simulink model "Collision_Test_Block_2020a"  (R2020a)
settings: Solver=ode4  StartTime=0.0  StopTime=15  FixedStep=0.001  RelTol=1e-6
values from neighbouring files (symbols this model uses):
  b = 200000    [Mini_Project.m]
  m = 80000    [Mini_Project.m]
  normal = 9.81*m    (= 784800)    [Mini_Project.m]
  u_kin = 0.05    [Mini_Project.m]
  u_st = 0.15    [Mini_Project.m]
libraries: simulink x3
settings Model: Creator=seano  LastModifiedBy=jackg
settings SolverCC: ZeroCrossAlgorithm=Adaptive
settings DebuggingCC: IgnoredZcDiagnostic=none  SFMachineParentedDataDiag=error

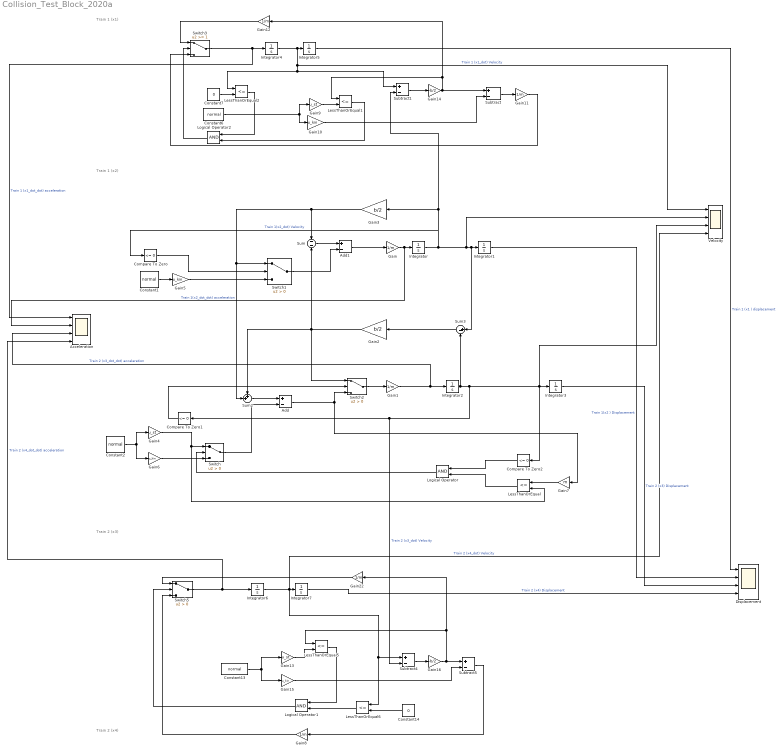
== system Collision_Test_Block_2020a ==
  note: Train 1 (x2)
  note: Train 1 (x1)
  note: Train 2 (x3)
  note: Train 2 (x4)
  Acceleration : Scope  NumInputPorts=4
  Add : Sum  Inputs=+-
  Add1 : Sum  Inputs=+-
  Compare To Zero : simulink/Logic and Bit Operations/Compare To Zero  relop=<=  OutDataTypeStr=boolean
  Compare To Zero1 : simulink/Logic and Bit Operations/Compare To Zero  relop=<=  OutDataTypeStr=boolean
  Compare To Zero2 : simulink/Logic and Bit Operations/Compare To Zero  relop=<=  OutDataTypeStr=boolean
  Constant{1..2,6,13} (4 alike) : Constant  Value=normal
  Constant14 : Constant  Value=0
  Constant7 : Constant  Value=0
  Displacement : Scope  NumInputPorts=4
  Gain{,1,8,11..12,22} (6 alike) : Gain  Gain=1/m
  Gain{5..6,10,15} (4 alike) : Gain  Gain=u_kin
  Gain13 : Gain  Gain=u_st
  Gain14 : Gain  Gain=-b/2
  Gain16 : Gain  Gain=-b/2
  Gain2 : Gain  Gain=b/2
  Gain3 : Gain  Gain=b/2
  Gain4 : Gain  Gain=u_st
  Gain7 : Gain  Gain=m
  Gain9 : Gain  Gain=u_st
  Integrator : Integrator  InitialCondition=13.9
  Integrator{1,3,5,7} (4 alike) : Integrator  InitialCondition=50
  Integrator2 : Integrator
  Integrator4 : Integrator  InitialCondition=13.9
  Integrator6 : Integrator
  LessThanOrEqual{,1..2,5..6} (5 alike) : RelationalOperator  Operator=<=  OutDataTypeStr=boolean  RndMeth=Simplest
  Logical Operator : Logic  AllPortsSameDT=off  OutDataTypeStr=boolean
  Logical Operator1 : Logic  AllPortsSameDT=off  OutDataTypeStr=boolean
  Logical Operator2 : Logic  AllPortsSameDT=off  OutDataTypeStr=boolean
  Subtract{,1,4..5} (4 alike) : Sum  Inputs=+-
  Sum : Sum  Inputs=--
  Sum2 : Sum  Inputs=++|
  Sum3 : Sum  Inputs=|+-
  Switch{,1..2,5} (4 alike) : Switch  Criteria=u2 > Threshold
  Switch3 : Switch  Threshold=1
  Velocity : Scope  NumInputPorts=4
  wires:
  Integrator/1 -> Subtract1/2, Gain3/1, Compare To Zero/1, Sum3/1, Integrator1/1, Velocity/2  "Train 1(x2_dot) Velocity"
  Integrator1/1 -> Displacement/2  "Train 1(x2 ) Displacement"
  Integrator3/1 -> Displacement/3  "Train 2 (x3) Displacement"
  Sum3/1 -> Gain2/1
  Gain3/1 -> Sum/1, Switch1/1, Sum2/2
  Constant2/1 -> Gain4/1, Gain6/1
  Constant1/1 -> Gain5/1
  Compare To Zero2/1 -> Logical Operator/1
  Logical Operator/1 -> Switch/2
  Gain6/1 -> Switch/3
  Gain7/1 -> LessThanOrEqual/1
  Gain4/1 -> LessThanOrEqual/2, Switch/1
  LessThanOrEqual/1 -> Logical Operator/2
  Switch/1 -> Add/2
  Add/1 -> Switch2/3, Gain7/1
  Gain/1 -> Acceleration/2, Integrator/1  "Train 1(x2_dot_dot) acceleration"
  Gain5/1 -> Switch1/3
  Compare To Zero/1 -> Switch1/2
  Switch1/1 -> Add1/2
  Switch2/1 -> Gain1/1
  Gain14/1 -> Subtract/1, Gain12/1, LessThanOrEqual1/1
  Compare To Zero1/1 -> Switch2/2
  Switch3/1 -> Acceleration/1, Integrator4/1  "Train 1 (x1_dot_dot) acceleration"
  Integrator4/1 -> Velocity/1, LessThanOrEqual2/1, Subtract1/1, Integrator5/1  "Train 1 (x1_dot) Velocity"
  Gain2/1 -> Switch2/1, Sum2/1, Sum/2
  Gain9/1 -> LessThanOrEqual1/2
  Constant6/1 -> Gain9/1, Gain10/1
  Constant7/1 -> LessThanOrEqual2/2
  Logical Operator2/1 -> Switch3/2
  Integrator5/1 -> Displacement/1  "Train 1 (x1 ) displacement"
  Subtract/1 -> Gain11/1
  Subtract1/1 -> Gain14/1
  Integrator2/1 -> Compare To Zero1/1, Subtract4/2, Compare To Zero2/1, Integrator3/1, Velocity/3, Sum3/2  "Train 2 (x3_dot) Velocity"
  Gain10/1 -> Subtract/2
  Gain11/1 -> Switch3/3
  Integrator6/1 -> Velocity/4, Integrator7/1, LessThanOrEqual6/1, Subtract4/1  "Train 2 (x4_dot) Velocity"
  Constant13/1 -> Gain13/1, Gain15/1
  Gain13/1 -> LessThanOrEqual5/2
  Constant14/1 -> LessThanOrEqual6/2
  Subtract4/1 -> Gain16/1
  Gain15/1 -> Subtract5/2
  Subtract5/1 -> Gain8/1
  Integrator7/1 -> Displacement/4  "Train 2 (x4) Displacement"
  LessThanOrEqual2/1 -> Logical Operator2/1
  LessThanOrEqual1/1 -> Logical Operator2/2
  Gain16/1 -> LessThanOrEqual5/1, Gain22/1, Subtract5/1
  Sum/1 -> Add1/1
  Switch5/1 -> Acceleration/4, Integrator6/1  "Train 2 (x4_dot_dot) acceleration"
  Gain8/1 -> Switch5/3
  LessThanOrEqual6/1 -> Logical Operator1/2
  LessThanOrEqual5/1 -> Logical Operator1/1
  Logical Operator1/1 -> Switch5/2
  Add1/1 -> Gain/1
  Gain12/1 -> Switch3/1
  Gain22/1 -> Switch5/1
  Sum2/1 -> Add/1
  Gain1/1 -> Acceleration/3, Integrator2/1  "Train 2 (x3_dot_dot) acceleration"
